simulink model "Regulation_02"  (R2022b)
settings: Solver=ode4  StartTime=0.0  StopTime=50  FixedStep=1e-3  MaxStep=1e-3  RelTol=1e-3
undefined symbols (not defined in the file or in its folder): p1, p2, p3, PR_k1, PR_k2, PR_k3, theta_d, tolerance_posture, v_sat, w_sat, x_d, y_d
libraries: dspsigops x3
settings Model: Creator=david  LastModifiedBy=david

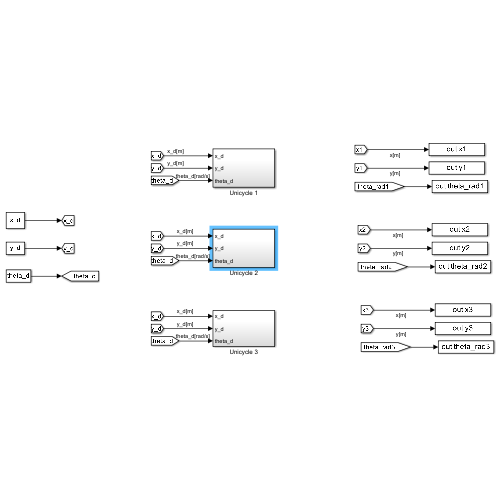
[thumbnail: Simulink's stored preview of the top-level diagram]
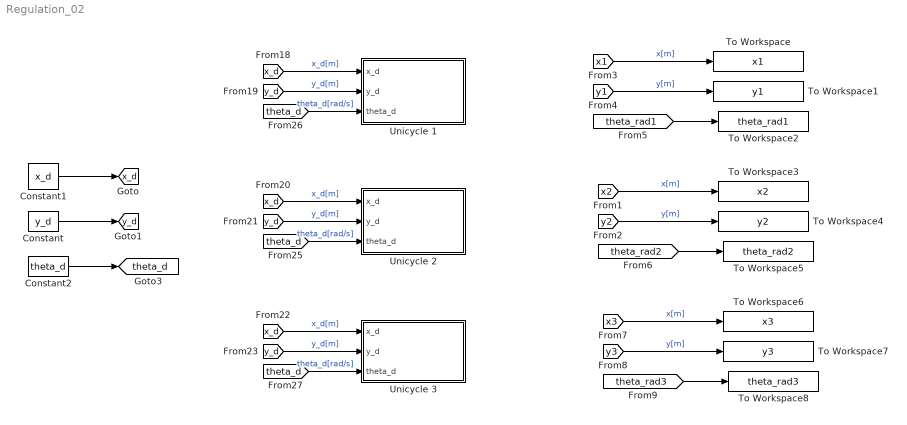
== system Regulation_02 ==
  Constant : Constant  Value=y_d
  Constant1 : Constant  Value=x_d
  Constant2 : Constant  Value=theta_d
  To Workspace : ToWorkspace  VariableName=x1  SaveFormat=Structure With Time  SampleTime=-1
  To Workspace1 : ToWorkspace  VariableName=y1  SaveFormat=Structure With Time  SampleTime=-1
  To Workspace2 : ToWorkspace  VariableName=theta_rad1  SaveFormat=Structure With Time  SampleTime=-1
  To Workspace3 : ToWorkspace  VariableName=x2  SaveFormat=Structure With Time  SampleTime=-1
  To Workspace4 : ToWorkspace  VariableName=y2  SaveFormat=Structure With Time  SampleTime=-1
  To Workspace5 : ToWorkspace  VariableName=theta_rad2  SaveFormat=Structure With Time  SampleTime=-1
  To Workspace6 : ToWorkspace  VariableName=x3  SaveFormat=Structure With Time  SampleTime=-1
  To Workspace7 : ToWorkspace  VariableName=y3  SaveFormat=Structure With Time  SampleTime=-1
  To Workspace8 : ToWorkspace  VariableName=theta_rad3  SaveFormat=Structure With Time  SampleTime=-1
  Unicycle 1 : Subsystem
  Unicycle 2 : Subsystem
  Unicycle 3 : Subsystem
  tag scope: theta_d=global, x_d=global, y_d=global
  wires:
  [x1] -> To Workspace/1  "x[m]"
  [y1] -> To Workspace1/1  "y[m]"
  [theta_rad1] -> To Workspace2/1
  [x2] -> To Workspace3/1  "x[m]"
  [y2] -> To Workspace4/1  "y[m]"
  [theta_rad2] -> To Workspace5/1
  [theta_rad3] -> To Workspace8/1
  [y3] -> To Workspace7/1  "y[m]"
  [x3] -> To Workspace6/1  "x[m]"
  Constant1/1 -> [x_d]
  Constant/1 -> [y_d]
  [x_d] -> Unicycle 1/1(x_d)  "x_d[m]"
  [y_d] -> Unicycle 1/2(y_d)  "y_d[m]"
  [y_d] -> Unicycle 2/2(y_d)  "y_d[m]"
  [x_d] -> Unicycle 2/1(x_d)  "x_d[m]"
  [y_d] -> Unicycle 3/2(y_d)  "y_d[m]"
  [x_d] -> Unicycle 3/1(x_d)  "x_d[m]"
  Constant2/1 -> [theta_d]
  [theta_d] -> Unicycle 2/3(theta_d)  "theta_d[rad/s]"
  [theta_d] -> Unicycle 1/3(theta_d)  "theta_d[rad/s]"
  [theta_d] -> Unicycle 3/3(theta_d)  "theta_d[rad/s]"

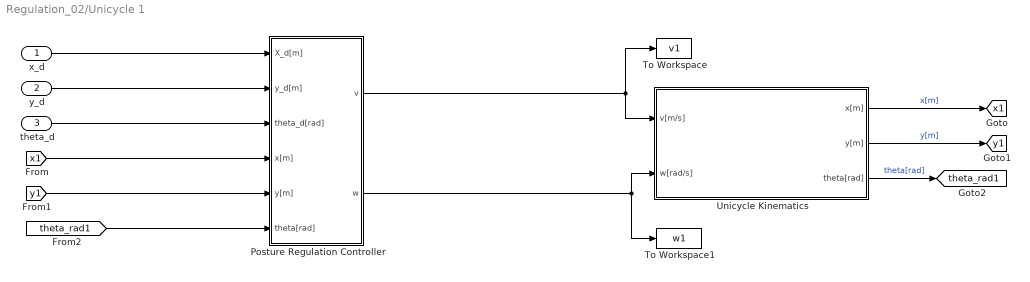
== system Regulation_02/Unicycle 1 ==
  x_d : Inport
  y_d : Inport  Port=2
  theta_d : Inport  Port=3
  Posture Regulation Controller : Subsystem
  To Workspace : ToWorkspace  VariableName=v1  SaveFormat=Structure With Time  SampleTime=-1
  To Workspace1 : ToWorkspace  VariableName=w1  SaveFormat=Structure With Time  SampleTime=-1
  Unicycle Kinematics : Subsystem
  tag scope: theta_rad1=global, x1=global, y1=global
  wires:
  Unicycle Kinematics/3(theta[rad]) -> [theta_rad1]  "theta[rad]"
  [y1] -> Posture Regulation Controller/5(y[m])
  [theta_rad1] -> Posture Regulation Controller/6(theta[rad])
  Unicycle Kinematics/2(y[m]) -> [y1]  "y[m]"
  [x1] -> Posture Regulation Controller/4(x[m])
  Unicycle Kinematics/1(x[m]) -> [x1]  "x[m]"
  x_d/1 -> Posture Regulation Controller/1(X_d[m])
  y_d/1 -> Posture Regulation Controller/2(y_d[m])
  Posture Regulation Controller/2(w) -> Unicycle Kinematics/2(w[rad/s]), To Workspace1/1
  Posture Regulation Controller/1(v) -> Unicycle Kinematics/1(v[m/s]), To Workspace/1
  theta_d/1 -> Posture Regulation Controller/3(theta_d[rad])

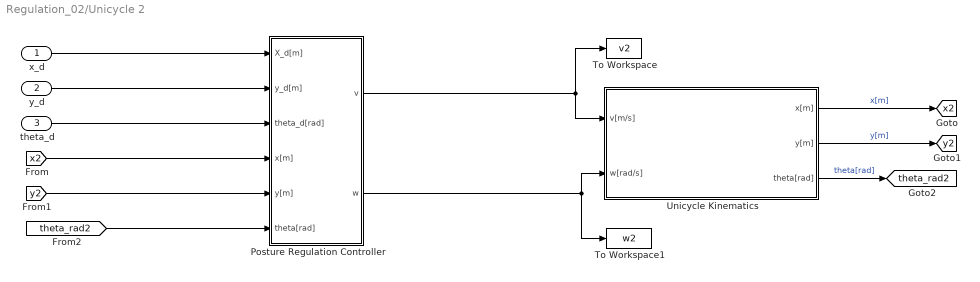
== system Regulation_02/Unicycle 2 ==
  x_d : Inport
  y_d : Inport  Port=2
  theta_d : Inport  Port=3
  Posture Regulation Controller : Subsystem
  To Workspace : ToWorkspace  VariableName=v2  SaveFormat=Structure With Time  SampleTime=-1
  To Workspace1 : ToWorkspace  VariableName=w2  SaveFormat=Structure With Time  SampleTime=-1
  Unicycle Kinematics : Subsystem
  tag scope: theta_rad2=global, x2=global, y2=global
  wires:
  Unicycle Kinematics/3(theta[rad]) -> [theta_rad2]  "theta[rad]"
  [y2] -> Posture Regulation Controller/5(y[m])
  [theta_rad2] -> Posture Regulation Controller/6(theta[rad])
  Unicycle Kinematics/2(y[m]) -> [y2]  "y[m]"
  [x2] -> Posture Regulation Controller/4(x[m])
  Unicycle Kinematics/1(x[m]) -> [x2]  "x[m]"
  x_d/1 -> Posture Regulation Controller/1(X_d[m])
  y_d/1 -> Posture Regulation Controller/2(y_d[m])
  Posture Regulation Controller/1(v) -> Unicycle Kinematics/1(v[m/s]), To Workspace/1
  theta_d/1 -> Posture Regulation Controller/3(theta_d[rad])
  Posture Regulation Controller/2(w) -> Unicycle Kinematics/2(w[rad/s]), To Workspace1/1

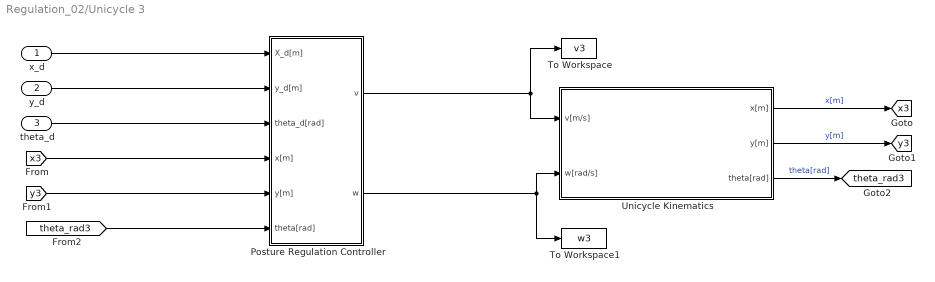
== system Regulation_02/Unicycle 3 ==
  x_d : Inport
  y_d : Inport  Port=2
  theta_d : Inport  Port=3
  Posture Regulation Controller : Subsystem
  To Workspace : ToWorkspace  VariableName=v3  SaveFormat=Structure With Time  SampleTime=-1
  To Workspace1 : ToWorkspace  VariableName=w3  SaveFormat=Structure With Time  SampleTime=-1
  Unicycle Kinematics : Subsystem
  tag scope: theta_rad3=global, x3=global, y3=global
  wires:
  Unicycle Kinematics/3(theta[rad]) -> [theta_rad3]  "theta[rad]"
  [y3] -> Posture Regulation Controller/5(y[m])
  [theta_rad3] -> Posture Regulation Controller/6(theta[rad])
  Unicycle Kinematics/2(y[m]) -> [y3]  "y[m]"
  [x3] -> Posture Regulation Controller/4(x[m])
  Unicycle Kinematics/1(x[m]) -> [x3]  "x[m]"
  x_d/1 -> Posture Regulation Controller/1(X_d[m])
  y_d/1 -> Posture Regulation Controller/2(y_d[m])
  Posture Regulation Controller/2(w) -> Unicycle Kinematics/2(w[rad/s]), To Workspace1/1
  Posture Regulation Controller/1(v) -> Unicycle Kinematics/1(v[m/s]), To Workspace/1
  theta_d/1 -> Posture Regulation Controller/3(theta_d[rad])

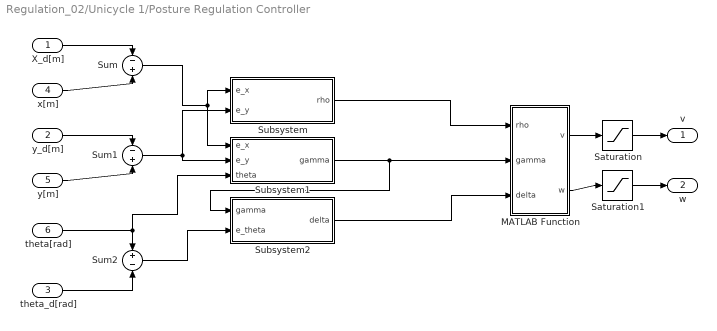
== system Regulation_02/Unicycle 1/Posture Regulation Controller ==
  X_d[m] : Inport
  y_d[m] : Inport  Port=2
  theta_d[rad] : Inport  Port=3
  x[m] : Inport  Port=4
  y[m] : Inport  Port=5
  theta[rad] : Inport  Port=6
  MATLAB Function : MATLAB Function  TreatAsAtomicUnit=on
  Saturation : Saturate  UpperLimit=v_sat  LowerLimit=-v_sat
  Saturation1 : Saturate  UpperLimit=w_sat  LowerLimit=-w_sat
  Subsystem : Subsystem
  Subsystem1 : Subsystem
  Subsystem2 : Subsystem
  Sum : Sum  Inputs=-+
  Sum1 : Sum  Inputs=-+
  Sum2 : Sum  Inputs=+-
  v : Outport
  w : Outport  Port=2
  wires:
  X_d[m]/1 -> Sum/1
  x[m]/1 -> Sum/2
  y_d[m]/1 -> Sum1/1
  y[m]/1 -> Sum1/2
  Sum1/1 -> Subsystem1/2(e_y), Subsystem/2(e_y)
  Sum2/1 -> Subsystem2/2(e_theta)
  Subsystem1/1(gamma) -> Subsystem2/1(gamma), MATLAB Function/2(gamma)
  Subsystem2/1(delta) -> MATLAB Function/3(delta)
  Subsystem/1(rho) -> MATLAB Function/1(rho)
  Sum/1 -> Subsystem1/1(e_x), Subsystem/1(e_x)
  MATLAB Function/1(v) -> Saturation/1
  MATLAB Function/2(w) -> Saturation1/1
  theta[rad]/1 -> Sum2/1, Subsystem1/3(theta)
  theta_d[rad]/1 -> Sum2/2
  Saturation/1 -> v/1
  Saturation1/1 -> w/1

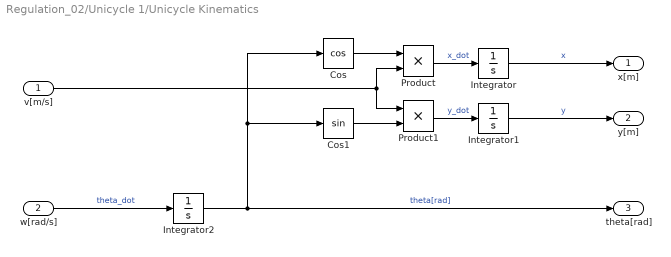
== system Regulation_02/Unicycle 1/Unicycle Kinematics ==
  v[m/s] : Inport
  w[rad/s] : Inport  Port=2
  Cos : Trigonometry  Operator=cos
  Cos1 : Trigonometry
  Integrator : Integrator  InitialCondition=p1(1)
  Integrator1 : Integrator  InitialCondition=p1(2)
  Integrator2 : Integrator  InitialCondition=p1(3)
  Product : Product
  Product1 : Product
  x[m] : Outport
  y[m] : Outport  Port=2
  theta[rad] : Outport  Port=3
  wires:
  Integrator/1 -> x[m]/1  "x"
  Integrator1/1 -> y[m]/1  "y"
  w[rad/s]/1 -> Integrator2/1  "theta_dot"
  Integrator2/1 -> Cos/1, Cos1/1, theta[rad]/1  "theta[rad]"
  Product/1 -> Integrator/1  "x_dot"
  Cos1/1 -> Product1/2
  Cos/1 -> Product/1
  v[m/s]/1 -> Product1/1, Product/2
  Product1/1 -> Integrator1/1  "y_dot"

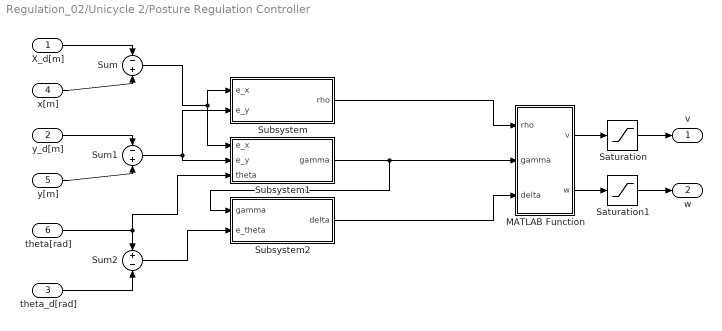
== system Regulation_02/Unicycle 2/Posture Regulation Controller ==
  X_d[m] : Inport
  y_d[m] : Inport  Port=2
  theta_d[rad] : Inport  Port=3
  x[m] : Inport  Port=4
  y[m] : Inport  Port=5
  theta[rad] : Inport  Port=6
  MATLAB Function : MATLAB Function  TreatAsAtomicUnit=on
  Saturation : Saturate  UpperLimit=v_sat  LowerLimit=-v_sat
  Saturation1 : Saturate  UpperLimit=w_sat  LowerLimit=-w_sat
  Subsystem : Subsystem
  Subsystem1 : Subsystem
  Subsystem2 : Subsystem
  Sum : Sum  Inputs=-+
  Sum1 : Sum  Inputs=-+
  Sum2 : Sum  Inputs=+-
  v : Outport
  w : Outport  Port=2
  wires:
  X_d[m]/1 -> Sum/1
  x[m]/1 -> Sum/2
  y_d[m]/1 -> Sum1/1
  y[m]/1 -> Sum1/2
  Sum1/1 -> Subsystem1/2(e_y), Subsystem/2(e_y)
  Sum2/1 -> Subsystem2/2(e_theta)
  Subsystem1/1(gamma) -> MATLAB Function/2(gamma), Subsystem2/1(gamma)
  Subsystem2/1(delta) -> MATLAB Function/3(delta)
  Subsystem/1(rho) -> MATLAB Function/1(rho)
  Sum/1 -> Subsystem1/1(e_x), Subsystem/1(e_x)
  MATLAB Function/1(v) -> Saturation/1
  MATLAB Function/2(w) -> Saturation1/1
  theta[rad]/1 -> Sum2/1, Subsystem1/3(theta)
  theta_d[rad]/1 -> Sum2/2
  Saturation/1 -> v/1
  Saturation1/1 -> w/1

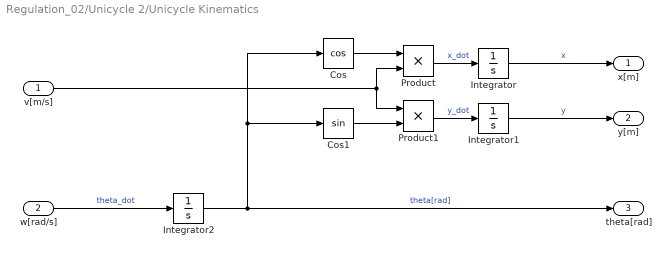
== system Regulation_02/Unicycle 2/Unicycle Kinematics ==
  v[m/s] : Inport
  w[rad/s] : Inport  Port=2
  Cos : Trigonometry  Operator=cos
  Cos1 : Trigonometry
  Integrator : Integrator  InitialCondition=p2(1)
  Integrator1 : Integrator  InitialCondition=p2(2)
  Integrator2 : Integrator  InitialCondition=p2(3)
  Product : Product
  Product1 : Product
  x[m] : Outport
  y[m] : Outport  Port=2
  theta[rad] : Outport  Port=3
  wires:
  Integrator/1 -> x[m]/1  "x"
  Integrator1/1 -> y[m]/1  "y"
  w[rad/s]/1 -> Integrator2/1  "theta_dot"
  Integrator2/1 -> Cos/1, Cos1/1, theta[rad]/1  "theta[rad]"
  Product/1 -> Integrator/1  "x_dot"
  Cos1/1 -> Product1/2
  Cos/1 -> Product/1
  v[m/s]/1 -> Product1/1, Product/2
  Product1/1 -> Integrator1/1  "y_dot"

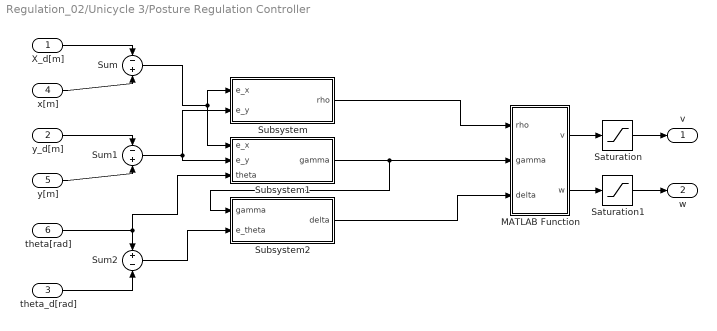
== system Regulation_02/Unicycle 3/Posture Regulation Controller ==
  X_d[m] : Inport
  y_d[m] : Inport  Port=2
  theta_d[rad] : Inport  Port=3
  x[m] : Inport  Port=4
  y[m] : Inport  Port=5
  theta[rad] : Inport  Port=6
  MATLAB Function : MATLAB Function  TreatAsAtomicUnit=on
  Saturation : Saturate  UpperLimit=v_sat  LowerLimit=-v_sat
  Saturation1 : Saturate  UpperLimit=w_sat  LowerLimit=-w_sat
  Subsystem : Subsystem
  Subsystem1 : Subsystem
  Subsystem2 : Subsystem
  Sum : Sum  Inputs=-+
  Sum1 : Sum  Inputs=-+
  Sum2 : Sum  Inputs=+-
  v : Outport
  w : Outport  Port=2
  wires:
  X_d[m]/1 -> Sum/1
  x[m]/1 -> Sum/2
  y_d[m]/1 -> Sum1/1
  y[m]/1 -> Sum1/2
  Sum1/1 -> Subsystem1/2(e_y), Subsystem/2(e_y)
  Sum2/1 -> Subsystem2/2(e_theta)
  Subsystem1/1(gamma) -> MATLAB Function/2(gamma), Subsystem2/1(gamma)
  Subsystem2/1(delta) -> MATLAB Function/3(delta)
  Subsystem/1(rho) -> MATLAB Function/1(rho)
  Sum/1 -> Subsystem1/1(e_x), Subsystem/1(e_x)
  MATLAB Function/1(v) -> Saturation/1
  MATLAB Function/2(w) -> Saturation1/1
  theta[rad]/1 -> Sum2/1, Subsystem1/3(theta)
  theta_d[rad]/1 -> Sum2/2
  Saturation/1 -> v/1
  Saturation1/1 -> w/1

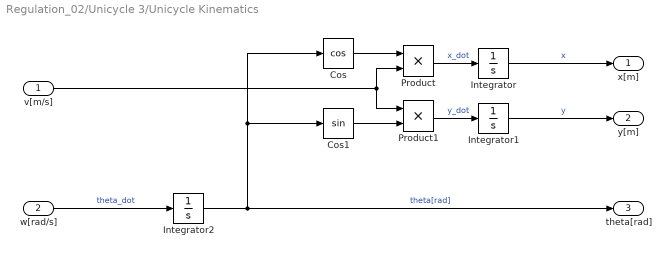
== system Regulation_02/Unicycle 3/Unicycle Kinematics ==
  v[m/s] : Inport
  w[rad/s] : Inport  Port=2
  Cos : Trigonometry  Operator=cos
  Cos1 : Trigonometry
  Integrator : Integrator  InitialCondition=p3(1)
  Integrator1 : Integrator  InitialCondition=p3(2)
  Integrator2 : Integrator  InitialCondition=p3(3)
  Product : Product
  Product1 : Product
  x[m] : Outport
  y[m] : Outport  Port=2
  theta[rad] : Outport  Port=3
  wires:
  Integrator/1 -> x[m]/1  "x"
  Integrator1/1 -> y[m]/1  "y"
  w[rad/s]/1 -> Integrator2/1  "theta_dot"
  Integrator2/1 -> Cos/1, Cos1/1, theta[rad]/1  "theta[rad]"
  Product/1 -> Integrator/1  "x_dot"
  Cos1/1 -> Product1/2
  Cos/1 -> Product/1
  v[m/s]/1 -> Product1/1, Product/2
  Product1/1 -> Integrator1/1  "y_dot"

== system Regulation_02/Unicycle 1/Posture Regulation Controller/Subsystem ==
  e_x : Inport
  e_y : Inport  Port=2
  Sqrt : Sqrt
  Square : Math  Operator=square
  Square1 : Math  Operator=square
  Sum : Sum
  rho : Outport
  wires:
  Sqrt/1 -> rho/1
  e_x/1 -> Square/1
  e_y/1 -> Square1/1
  Sum/1 -> Sqrt/1
  Square/1 -> Sum/1
  Square1/1 -> Sum/2

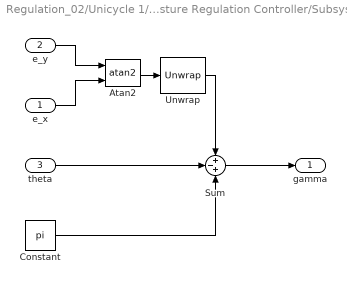
== system Regulation_02/Unicycle 1/Posture Regulation Controller/Subsystem1 ==
  e_x : Inport
  e_y : Inport  Port=2
  theta : Inport  Port=3
  Atan2 : Trigonometry  Operator=atan2
  Constant : Constant  Value=pi
  Sum : Sum  Inputs=+-+
  Unwrap : dspsigops/Unwrap  tol=pi  InputProcessing=Columns as channels (frame based)  running=off
  gamma : Outport
  wires:
  e_x/1 -> Atan2/2
  e_y/1 -> Atan2/1
  theta/1 -> Sum/2
  Sum/1 -> gamma/1
  Atan2/1 -> Unwrap/1
  Constant/1 -> Sum/3
  Unwrap/1 -> Sum/1

== system Regulation_02/Unicycle 1/Posture Regulation Controller/Subsystem2 ==
  gamma : Inport
  e_theta : Inport  Port=2
  Sum : Sum
  delta : Outport
  wires:
  e_theta/1 -> Sum/2
  Sum/1 -> delta/1
  gamma/1 -> Sum/1

== system Regulation_02/Unicycle 2/Posture Regulation Controller/Subsystem ==
  e_x : Inport
  e_y : Inport  Port=2
  Sqrt : Sqrt
  Square : Math  Operator=square
  Square1 : Math  Operator=square
  Sum : Sum
  rho : Outport
  wires:
  Sqrt/1 -> rho/1
  e_x/1 -> Square/1
  e_y/1 -> Square1/1
  Sum/1 -> Sqrt/1
  Square/1 -> Sum/1
  Square1/1 -> Sum/2

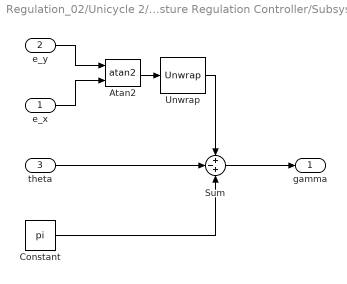
== system Regulation_02/Unicycle 2/Posture Regulation Controller/Subsystem1 ==
  e_x : Inport
  e_y : Inport  Port=2
  theta : Inport  Port=3
  Atan2 : Trigonometry  Operator=atan2
  Constant : Constant  Value=pi
  Sum : Sum  Inputs=+-+
  Unwrap : dspsigops/Unwrap  tol=pi  InputProcessing=Columns as channels (frame based)  running=off
  gamma : Outport
  wires:
  e_x/1 -> Atan2/2
  e_y/1 -> Atan2/1
  theta/1 -> Sum/2
  Sum/1 -> gamma/1
  Atan2/1 -> Unwrap/1
  Constant/1 -> Sum/3
  Unwrap/1 -> Sum/1

== system Regulation_02/Unicycle 2/Posture Regulation Controller/Subsystem2 ==
  gamma : Inport
  e_theta : Inport  Port=2
  Sum : Sum
  delta : Outport
  wires:
  e_theta/1 -> Sum/2
  Sum/1 -> delta/1
  gamma/1 -> Sum/1

== system Regulation_02/Unicycle 3/Posture Regulation Controller/Subsystem ==
  e_x : Inport
  e_y : Inport  Port=2
  Sqrt : Sqrt
  Square : Math  Operator=square
  Square1 : Math  Operator=square
  Sum : Sum
  rho : Outport
  wires:
  Sqrt/1 -> rho/1
  e_x/1 -> Square/1
  e_y/1 -> Square1/1
  Sum/1 -> Sqrt/1
  Square/1 -> Sum/1
  Square1/1 -> Sum/2

== system Regulation_02/Unicycle 3/Posture Regulation Controller/Subsystem1 ==
  e_x : Inport
  e_y : Inport  Port=2
  theta : Inport  Port=3
  Atan2 : Trigonometry  Operator=atan2
  Constant : Constant  Value=pi
  Sum : Sum  Inputs=+-+
  Unwrap : dspsigops/Unwrap  tol=pi  InputProcessing=Columns as channels (frame based)  running=off
  gamma : Outport
  wires:
  e_x/1 -> Atan2/2
  e_y/1 -> Atan2/1
  theta/1 -> Sum/2
  Sum/1 -> gamma/1
  Atan2/1 -> Unwrap/1
  Constant/1 -> Sum/3
  Unwrap/1 -> Sum/1

== system Regulation_02/Unicycle 3/Posture Regulation Controller/Subsystem2 ==
  gamma : Inport
  e_theta : Inport  Port=2
  Sum : Sum
  delta : Outport
  wires:
  e_theta/1 -> Sum/2
  Sum/1 -> delta/1
  gamma/1 -> Sum/1

== matlab function Regulation_02/Unicycle 2/Posture Regulation Controller/MATLAB Function ==
  data: rho input; v output; w output; gamma input; delta input; PR_k1 parameter; PR_k2 parameter; PR_k3 parameter; tolerance_posture parameter
function [v,w] = fcn(rho, gamma, delta, PR_k1, PR_k2, PR_k3, tolerance_posture)

if abs(rho)<tolerance_posture
    v=0;
    w=0;
else
    v=PR_k1*rho*cos(gamma);
    w=PR_k2*gamma+PR_k1*(cos(gamma)*sin(gamma))/gamma*(gamma+PR_k3*delta);
end

== matlab function Regulation_02/Unicycle 3/Posture Regulation Controller/MATLAB Function ==
  data: rho input; v output; w output; gamma input; delta input; PR_k1 parameter; PR_k2 parameter; PR_k3 parameter; tolerance_posture parameter
function [v,w] = fcn(rho, gamma, delta, PR_k1, PR_k2, PR_k3, tolerance_posture)

if abs(rho)<tolerance_posture
    v=0;
    w=0;
else
    v=PR_k1*rho*cos(gamma);
    w=PR_k2*gamma+PR_k1*(cos(gamma)*sin(gamma))/gamma*(gamma+PR_k3*delta);
end

== matlab function Regulation_02/Unicycle 1/Posture Regulation Controller/MATLAB Function ==
  data: rho input; v output; w output; gamma input; delta input; PR_k1 parameter; PR_k2 parameter; PR_k3 parameter; tolerance_posture parameter
function [v,w] = fcn(rho, gamma, delta, PR_k1, PR_k2, PR_k3, tolerance_posture)

if abs(rho)<tolerance_posture
    v=0;
    w=0;
else
    v=PR_k1*rho*cos(gamma);
    w=PR_k2*gamma+PR_k1*(cos(gamma)*sin(gamma))/gamma*(gamma+PR_k3*delta);
end
